simulink model "FinalHTTRModel"  (R2025b)
settings: Solver=ode15s  StartTime=0.0  StopTime=250  MaxStep=0.01  RelTol=1e-3
settings Model: Creator=jf923  LastModifiedBy=dm1124
settings DebuggingCC: AlgebraicLoopMsg=none

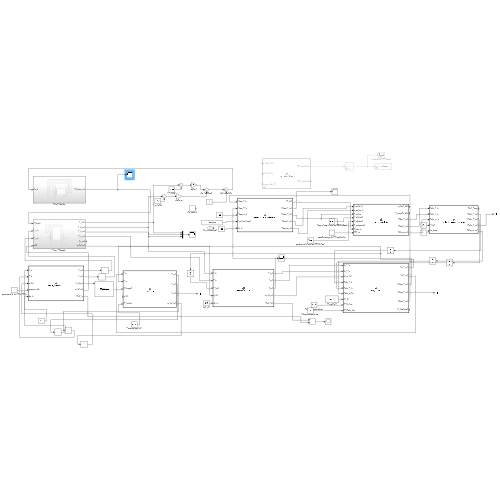
[thumbnail: Simulink's stored preview of the top-level diagram]
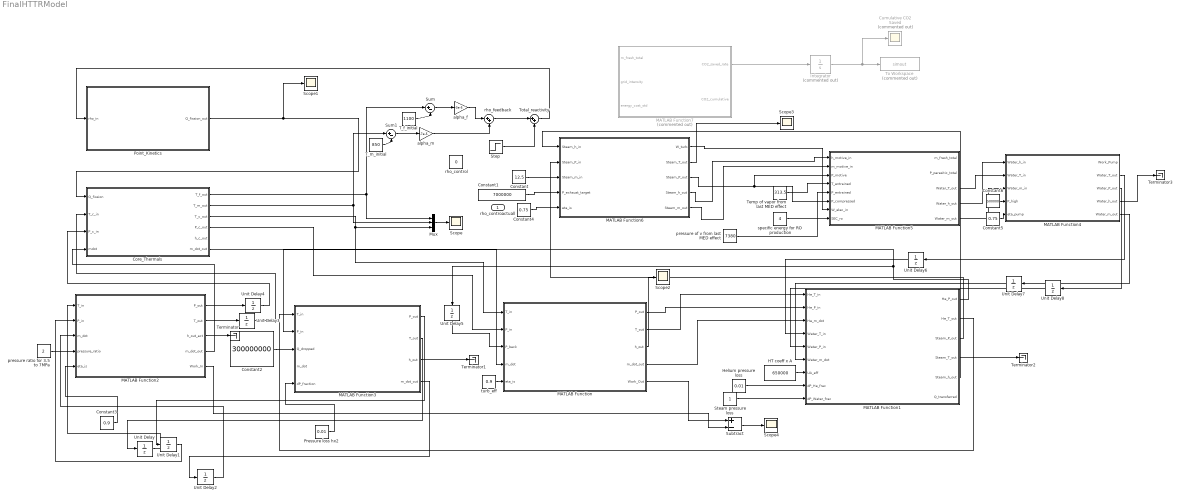
== system FinalHTTRModel ==
  rho_controactuall : Inport
  Constant : Constant  Value=12.5
  Constant1 : Constant  Value=7000000
  Constant2 : Constant  Value=300000000
  Constant3 : Constant  Value=0.9
  Constant4 : Constant  Value=0.75
  Constant5 : Constant  Value=0.75
  Constant6 : Constant  Value=500000
  Core_Thermals : Subsystem
  Cumulative CO2 Saved : Scope  Commented=on
      settings: DataLoggingVariableName=ScopeData3
  HT coeff x A : Constant  Value=650000
  Helium pressure loss : Constant  Value=0.01
  Integrator : Integrator  Commented=on
  MATLAB Function : MATLAB Function  TreatAsAtomicUnit=on  SystemSampleTime=0.1
  MATLAB Function1 : MATLAB Function  TreatAsAtomicUnit=on  SystemSampleTime=0.01
  MATLAB Function2 : MATLAB Function  TreatAsAtomicUnit=on
  MATLAB Function3 : MATLAB Function  TreatAsAtomicUnit=on
  MATLAB Function4 : MATLAB Function  TreatAsAtomicUnit=on
  MATLAB Function5 : MATLAB Function  TreatAsAtomicUnit=on
  MATLAB Function6 : MATLAB Function  TreatAsAtomicUnit=on
  MATLAB Function7 : MATLAB Function  Commented=on  TreatAsAtomicUnit=on
  Mux : Mux  Inputs=3
  Point_Kinetics : Subsystem
  Pressure loss hx2 : Constant  Value=0.01
  Scope{,1..4} (5 alike) : Scope
      Scope settings: ActiveDisplayYMinimum=-2.493928501622884  ActiveDisplayYMaximum=3.810317674067397
      Scope1 settings: ActiveDisplayYMinimum=-6.0368369547673821E+8  ActiveDisplayYMaximum=1.471994974635426E+9
      Scope2 settings: ActiveDisplayYMinimum=2.3690004673826769E+6  ActiveDisplayYMaximum=7.514541427479011E+6  DataLoggingVariableName=ScopeData2
      Scope3 settings: ActiveDisplayYMinimum=344.58792109090257  ActiveDisplayYMaximum=344.7374195032  DataLoggingVariableName=ScopeData5
      Scope4 settings: ActiveDisplayYMinimum=-1.4989347096918812E+9  ActiveDisplayYMaximum=2.98594671527647E+9  DataLoggingVariableName=ScopeData4
  Steam pressure loss : Constant
  Step : Step  Time=100  After=0.001  SampleTime=0
  Subtract : Sum  Inputs=+-
  Sum : Sum  Inputs=|+-
  Sum1 : Sum  Inputs=|+-
  T_f_initial : Constant  Value=1100
  T_m_initial : Constant  Value=850
  Temp of vapor from last MED effect : Constant  Value=313.5
  Terminator{,1..3} (4 alike) : Terminator
  To Workspace : ToWorkspace  Commented=on  VariableName=simout  SaveFormat=Timeseries  SampleTime=-1
  Total_reactivity : Sum  Inputs=|++
  Unit Delay : UnitDelay  InitialCondition=300  SampleTime=-1  HasFrameUpgradeWarning=on
  Unit Delay1 : UnitDelay  InitialCondition=3.5e6  SampleTime=-1  HasFrameUpgradeWarning=on
  Unit Delay2 : UnitDelay  InitialCondition=1000  SampleTime=-1  HasFrameUpgradeWarning=on
  Unit Delay3 : UnitDelay  InitialCondition=500  SampleTime=-1  HasFrameUpgradeWarning=on
  Unit Delay4 : UnitDelay  InitialCondition=7000000  SampleTime=0.01  HasFrameUpgradeWarning=on
  Unit Delay5 : UnitDelay  InitialCondition=7000000  SampleTime=-1  HasFrameUpgradeWarning=on
  Unit Delay6 : UnitDelay  InitialCondition=343  SampleTime=-1  HasFrameUpgradeWarning=on
  Unit Delay7 : UnitDelay  InitialCondition=100  SampleTime=-1  HasFrameUpgradeWarning=on
  Unit Delay8 : UnitDelay  InitialCondition=7000000  SampleTime=-1  HasFrameUpgradeWarning=on
  alpha_f : Gain  Gain=-3e-5
  alpha_m : Gain  Gain=-7e-5
  pressure of v from last MED effect : Constant  Value=7380
  pressure ratio for 3.5 to 7MPa : Constant  Value=2
  rho_control : Constant  Value=0
  rho_feedback : Sum  Inputs=|++
  specific energy for RO production : Constant  Value=4
  turb_eff : Constant  Value=0.9
  wires:
  Point_Kinetics/1(Q_fission_out) -> Core_Thermals/1(Q_fission), Scope1/1
  MATLAB Function/2(T_out) -> MATLAB Function1/1(He_T_in)
  Core_Thermals/1(T_f_out) -> Mux/1, Sum/1
  Core_Thermals/2(T_m_out) -> Mux/2, Sum1/1
  Core_Thermals/3(T_c_out) -> MATLAB Function/1(T_in), Mux/3
  T_f_initial/1 -> Sum/2
  T_m_initial/1 -> Sum1/2
  Sum/1 -> alpha_f/1
  Sum1/1 -> alpha_m/1
  alpha_f/1 -> rho_feedback/1
  alpha_m/1 -> rho_feedback/2
  rho_feedback/1 -> Total_reactivity/1
  Total_reactivity/1 -> Point_Kinetics/1(rho_in)
  Mux/1 -> Scope/1
  Step/1 -> Total_reactivity/2
  turb_eff/1 -> MATLAB Function/5(eta_is)
  MATLAB Function/3(h_out) -> Scope2/1
  MATLAB Function/1(P_out) -> MATLAB Function1/2(He_P_in)
  MATLAB Function/4(m_dot_out) -> MATLAB Function1/3(He_m_dot)
  MATLAB Function2/1(P_out) -> Unit Delay4/1
  Core_Thermals/4(P_c_out) -> MATLAB Function/2(P_in)
  MATLAB Function2/4(m_dot_out) -> Core_Thermals/4(mdot)
  MATLAB Function2/2(T_out) -> Unit Delay3/1
  Core_Thermals/6(m_dot_out) -> MATLAB Function/4(m_dot)
  MATLAB Function1/1(He_P_out) -> MATLAB Function3/2(P_in), Unit Delay5/1
  MATLAB Function1/2(He_T_out) -> MATLAB Function3/1(T_in)
  MATLAB Function1/5(Steam_h_out) -> MATLAB Function6/1(Steam_h_in)
  Constant3/1 -> MATLAB Function2/5(eta_is)
  Helium pressure loss/1 -> MATLAB Function1/8(dP_He_frac)
  MATLAB Function2/5(Work_In) -> Subtract/2
  MATLAB Function/5(Work_Out) -> Subtract/1
  Subtract/1 -> Scope4/1
  MATLAB Function2/3(h_out_act) -> Terminator/1
  MATLAB Function3/3(h_out) -> Terminator1/1
  MATLAB Function1/4(Steam_T_out) -> Terminator2/1
  Constant2/1 -> MATLAB Function3/3(Q_dropped)
  Pressure loss hx2/1 -> MATLAB Function3/5(dP_fraction)
  pressure ratio for 3.5 to 7MPa/1 -> MATLAB Function2/4(pressure_ratio)
  MATLAB Function3/2(T_out) -> Unit Delay/1
  Unit Delay/1 -> MATLAB Function2/1(T_in)
  MATLAB Function3/1(P_out) -> Unit Delay1/1
  MATLAB Function3/4(m_dot_out) -> Unit Delay2/1
  Unit Delay1/1 -> MATLAB Function2/2(P_in)
  Unit Delay2/1 -> MATLAB Function2/3(m_dot)
  Unit Delay3/1 -> Core_Thermals/2(T_c_in)
  Unit Delay4/1 -> Core_Thermals/3(P_c_in)
  Unit Delay5/1 -> MATLAB Function/3(P_back)
  MATLAB Function7/1(CO2_saved_rate) -> Integrator/1
  HT coeff x A/1 -> MATLAB Function1/7(UA_eff)
  Steam pressure loss/1 -> MATLAB Function1/9(dP_Water_frac)
  MATLAB Function5/3(Water_T_out) -> MATLAB Function4/2(Water_T_in)
  MATLAB Function5/5(Water_m_out) -> MATLAB Function4/3(Water_m_in)
  MATLAB Function1/3(Steam_P_out) -> MATLAB Function6/2(Steam_P_in)
  MATLAB Function6/4(Steam_h_out) -> MATLAB Function5/1(h_motive_in)
  MATLAB Function6/5(Steam_m_out) -> MATLAB Function5/2(m_motive_in)
  MATLAB Function6/1(W_turb) -> MATLAB Function5/7(W_elec_in)
  MATLAB Function6/3(Steam_P_out) -> MATLAB Function5/6(P_compressed), MATLAB Function5/3(P_motive)
  Temp of vapor from last MED effect/1 -> MATLAB Function5/4(T_entrained)
  pressure of v from last MED effect/1 -> MATLAB Function5/5(P_entrained)
  specific energy for RO production/1 -> MATLAB Function5/8(SEC_ro)
  MATLAB Function4/3(Water_P_out) -> Unit Delay8/1
  MATLAB Function5/4(Water_h_out) -> MATLAB Function4/1(Water_h_in)
  MATLAB Function4/4(Water_h_out) -> Terminator3/1
  MATLAB Function4/2(Water_T_out) -> Unit Delay6/1
  MATLAB Function4/5(Water_m_out) -> Unit Delay7/1
  Integrator/1 -> Cumulative CO2 Saved/1, To Workspace/1
  Unit Delay6/1 -> MATLAB Function1/4(Water_T_in)
  Unit Delay7/1 -> MATLAB Function1/6(Water_m_dot)
  Unit Delay8/1 -> MATLAB Function1/5(Water_P_in)
  Constant/1 -> MATLAB Function6/3(Steam_m_in)
  Constant1/1 -> MATLAB Function6/4(P_exhaust_target)
  Constant4/1 -> MATLAB Function6/5(eta_is)
  Constant5/1 -> MATLAB Function4/5(eta_pump)
  Constant6/1 -> MATLAB Function4/4(P_high)
  MATLAB Function6/2(Steam_T_out) -> Scope3/1

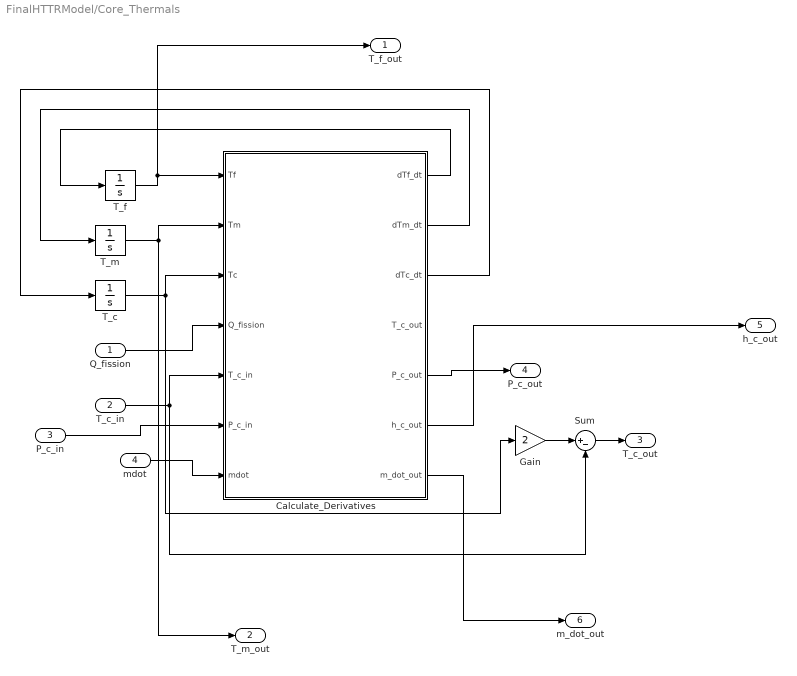
== system FinalHTTRModel/Core_Thermals ==
  Q_fission : Inport
  T_c_in : Inport  Port=2
  P_c_in : Inport  Port=3
  mdot : Inport  Port=4
  Calculate_Derivatives : MATLAB Function  TreatAsAtomicUnit=on
  Gain : Gain  Gain=2
  Sum : Sum  Inputs=|+-
  T_c : Integrator  InitialCondition=550
  T_f : Integrator  InitialCondition=600
  T_m : Integrator  InitialCondition=600
  T_f_out : Outport
  T_m_out : Outport  Port=2
  T_c_out : Outport  Port=3
  P_c_out : Outport  Port=4
  h_c_out : Outport  Port=5
  m_dot_out : Outport  Port=6
  wires:
  T_f/1 -> T_f_out/1, Calculate_Derivatives/1(Tf)
  T_m/1 -> T_m_out/1, Calculate_Derivatives/2(Tm)
  T_c/1 -> Gain/1, Calculate_Derivatives/3(Tc)
  Calculate_Derivatives/1(dTf_dt) -> T_f/1
  Q_fission/1 -> Calculate_Derivatives/4(Q_fission)
  T_c_in/1 -> Sum/2, Calculate_Derivatives/5(T_c_in)
  mdot/1 -> Calculate_Derivatives/7(mdot)
  Gain/1 -> Sum/1
  Sum/1 -> T_c_out/1
  Calculate_Derivatives/2(dTm_dt) -> T_m/1
  Calculate_Derivatives/3(dTc_dt) -> T_c/1
  P_c_in/1 -> Calculate_Derivatives/6(P_c_in)
  Calculate_Derivatives/5(P_c_out) -> P_c_out/1
  Calculate_Derivatives/6(h_c_out) -> h_c_out/1
  Calculate_Derivatives/7(m_dot_out) -> m_dot_out/1

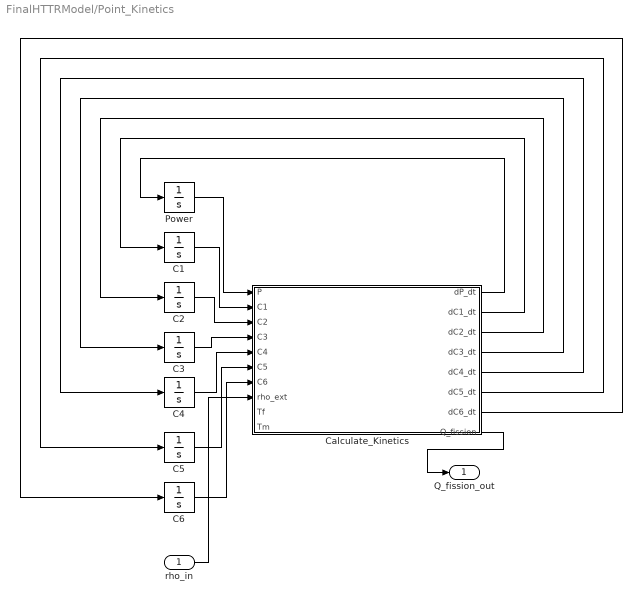
== system FinalHTTRModel/Point_Kinetics ==
  rho_in : Inport
  C1 : Integrator  InitialCondition=32.6371
  C2 : Integrator  InitialCondition=48.8496
  C3 : Integrator  InitialCondition=19.8245
  C4 : Integrator  InitialCondition=16.2791
  C5 : Integrator  InitialCondition=3.1685
  C6 : Integrator  InitialCondition=0.2093
  Calculate_Kinetics : MATLAB Function  TreatAsAtomicUnit=on
  Power : Integrator  InitialCondition=1
  Q_fission_out : Outport
  wires:
  Power/1 -> Calculate_Kinetics/1(P)
  C1/1 -> Calculate_Kinetics/2(C1)
  C2/1 -> Calculate_Kinetics/3(C2)
  C3/1 -> Calculate_Kinetics/4(C3)
  C4/1 -> Calculate_Kinetics/5(C4)
  C5/1 -> Calculate_Kinetics/6(C5)
  C6/1 -> Calculate_Kinetics/7(C6)
  rho_in/1 -> Calculate_Kinetics/8(rho_ext)
  Calculate_Kinetics/1(dP_dt) -> Power/1
  Calculate_Kinetics/2(dC1_dt) -> C1/1
  Calculate_Kinetics/3(dC2_dt) -> C2/1
  Calculate_Kinetics/4(dC3_dt) -> C3/1
  Calculate_Kinetics/5(dC4_dt) -> C4/1
  Calculate_Kinetics/6(dC5_dt) -> C5/1
  Calculate_Kinetics/7(dC6_dt) -> C6/1
  Calculate_Kinetics/8(Q_fission) -> Q_fission_out/1

== matlab function FinalHTTRModel/MATLAB Function2 ==
  data: T_in input; P_out output; T_out output; P_in input; m_dot input; pressure_ratio input; eta_is input; h_out_act output; m_dot_out output; Work_In output
function [P_out, T_out, h_out_act, m_dot_out, Work_In] = helium_compressor(T_in, P_in, m_dot, pressure_ratio, eta_is)
    coder.extrinsic('py.CoolProp.CoolProp.PropsSI');
    P_out = 0.0; T_out = 0.0; h_out_act = 0.0; m_dot_out = 0.0; Work_In = 0.0;
    fluid = 'Helium';
    
    if T_in <= 10 || P_in <= 1000000 || m_dot <= 0
        P_out = double(P_in); T_out = double(T_in); m_dot_out = double(m_dot);
    else
        h_in = 0.0;
        s_in = 0.0;
        h_out_s = 0.0;
        T_out_calc = 0.0;

        h_in_val = py.CoolProp.CoolProp.PropsSI('H', 'T', double(T_in), 'P', double(P_in), fluid);
        h_in = double(h_in_val);
        
        s_in_val = py.CoolProp.CoolProp.PropsSI('S', 'T', double(T_in), 'P', double(P_in), fluid);
        s_in = double(s_in_val);
        
        P_out_target = double(P_in) * double(pressure_ratio);
        
        h_s_val = py.CoolProp.CoolProp.PropsSI('H', 'S', s_in, 'P', P_out_target, fluid);
        h_out_s = double(h_s_val);
        
        h_out_act_val = h_in + (h_out_s - h_in) / double(eta_is);
        h_out_act = double(h_out_act_val);
        
        T_out_val = py.CoolProp.CoolProp.PropsSI('T', 'H', h_out_act, 'P', P_out_target, fluid);
        T_out = double(T_out_val);
        
        P_out = P_out_target;
        m_dot_out = double(m_dot);
        Work_In = double(m_dot) * (h_out_act - h_in);
    end
end

== matlab function FinalHTTRModel/MATLAB Function3 ==
  data: T_in input; P_out output; P_in input; Q_dropped input; m_dot input; dP_fraction input; T_out output; h_out output; m_dot_out output
function [P_out, T_out, h_out, m_dot_out] = helium_hx(T_in, P_in, Q_dropped, m_dot, dP_fraction)
    coder.extrinsic('py.CoolProp.CoolProp.PropsSI');
    P_out = 0.0; T_out = 0.0; h_out = 0.0; m_dot_out = 0.0;
    fluid = 'Helium';
    
    if T_in <= 10 || P_in <= 1000 || m_dot <= 0
        P_out = double(P_in); T_out = double(T_in); m_dot_out = double(m_dot);
    else
        h_in = 0.0;
        T_out_val = 0.0;

        h_in_raw = py.CoolProp.CoolProp.PropsSI('H', 'T', double(T_in), 'P', double(P_in), fluid);
        h_in = double(h_in_raw);
        
        h_out = h_in - (double(Q_dropped) / double(m_dot));
        
        P_out = double(P_in) * (1.0 - double(dP_fraction));
        
        T_out_raw = py.CoolProp.CoolProp.PropsSI('T', 'H', h_out, 'P', P_out, fluid);
        T_out = double(T_out_raw);
        
        m_dot_out = double(m_dot);
    end
end

== matlab function FinalHTTRModel/MATLAB Function4 ==
  data: Work_Pump output; Water_h_in input; Water_T_in input; Water_T_out output; Water_m_in input; P_high input; eta_pump input; Water_P_out output; Water_h_out output; Water_m_out output
function [Work_Pump, Water_T_out, Water_P_out, Water_h_out, Water_m_out] = feedwater_pump_measured(Water_h_in, Water_T_in, Water_m_in, P_high, eta_pump)
    % Declare extrinsic functions for CoolProp
    coder.extrinsic('py.CoolProp.CoolProp.PropsSI');
    fluid = 'Water';
    
    % 1. Pre-initialize variables as doubles to satisfy the Coder
    rho_water = 0.0;
    Work_Pump = 0.0;
    Water_h_out = 0.0;
    Water_T_out = 0.0;
    
    % 2. Calculate Density based on incoming temperature
    % Use an intermediate variable for the mxArray before casting to double
    rho_mx = py.CoolProp.CoolProp.PropsSI('D', 'T', double(Water_T_in), 'P', 31000, fluid);
    rho_water = double(rho_mx);
    
    % 3. Pressurization and Work calculation
    delta_P = double(P_high) - 31000;
    % Ensure all components are treated as numeric doubles
    Work_Pump = (double(Water_m_in) * delta_P) / (rho_water * double(eta_pump));
    
    % 4. Outlet State Assignment
    Water_P_out = double(P_high);
    Water_m_out = double(Water_m_in);
    
    % 5. Calculate Enthalpy increase
    % Work_Pump is now a confirmed double, allowing math operations
    Water_h_out = double(Water_h_in) + (Work_Pump / double(Water_m_in));
    
    % Final CoolProp call for temperature
    T_out_mx = py.CoolProp.CoolProp.PropsSI('T', 'H', Water_h_out, 'P', Water_P_out, fluid);
    Water_T_out = double(T_out_mx);
end

== matlab function FinalHTTRModel/MATLAB Function5 ==
  data: h_motive_in input; m_fresh_total output; m_motive_in input; P_motive input; T_entrained input; P_entrained input; P_compressed input; W_elec_in input; SEC_ro input; P_parasitic_total output; Water_T_out output; Water_h_out output; Water_m_out output
function [m_fresh_total, P_parasitic_total, Water_T_out, Water_h_out, Water_m_out] = hybrid_desal_tvc(h_motive_in, m_motive_in, P_motive, T_entrained, P_entrained, P_compressed, W_elec_in, SEC_ro)
    % h_motive_in: Enthalpy from LP Turbine outlet (Motive Steam)
    % m_motive_in: Steam flow from Turbine (kg/s)
    % T_entrained/P_entrained: Conditions of vapor from last MED effect
    
    coder.extrinsic('py.CoolProp.CoolProp.PropsSI');
    
    Water_h_out = 0;
    % 1. TVC Entrainment Ratio (Ra)
    % Ra = flow rate of motive steam / flow rate of entrained vapor
    % Using the Power (1994) simplified correlation provided in text
    PCF = 3e-7 * P_motive + 0.95; % Pressure Correction Factor
    TCF = 1.0; % Temp Correction Factor (Simplified for Phase 1)
    Cr = P_compressed / P_entrained; % Compression Ratio
    
    % Ra calculation (Semi-empirical model)
    Ra = 0.29 * (Cr^1.19) / (PCF * TCF); 
    m_entrained = m_motive_in / Ra;
    
    % 2. MED Performance (Thermal)
    % Total heating steam = motive + entrained
    m_heating_steam = m_motive_in + m_entrained;
    % GOR is typically higher for TVC (e.g., 10-14)
    GOR_tvc = 12.0; 
    m_fresh_med = m_heating_steam * GOR_tvc; 

    % 3. RO Process (Electrical)
    m_fresh_ro = W_elec_in / (SEC_ro * 3600); % J/kg conversion

    % 4. Output State for Closed-Loop (To Pump/HRSG)
    % The motive steam and entrained vapor condense into liquid water
    Water_m_out = m_motive_in; % Mass balance of the loop fluid
    Water_T_out = 343.15; % 70 C return temp (saturated liquid)
    Water_h_out = double(py.CoolProp.CoolProp.PropsSI('H', 'T', Water_T_out, 'P', P_compressed, 'Water'));
    
    % 5. System Totals
    m_fresh_total = m_fresh_med + m_fresh_ro;
    P_parasitic_total = W_elec_in; % Load for RO Pumps
end

== matlab function FinalHTTRModel/MATLAB Function6 ==
  data: Steam_h_in input; W_turb output; Steam_P_in input; Steam_m_in input; P_exhaust_target input; eta_is input; Steam_T_out output; Steam_P_out output; Steam_h_out output; Steam_m_out output
function [W_turb, Steam_T_out, Steam_P_out, Steam_h_out, Steam_m_out] = steam_turbine_measured(Steam_h_in, Steam_P_in, Steam_m_in, P_exhaust_target, eta_is)
    % Declare extrinsic functions
    coder.extrinsic('py.CoolProp.CoolProp.PropsSI');
    
    % 1. Initialize variables to define them as double scalars for the Coder
    fluid = 'Water';
    s_in = 0; 
    h_out_s = 0;
    T_out_val = 0;
    Steam_T_out = 0;
    
    % 2. Inlet Entropy calculation
    % We call the function and immediately cast the output to double
    s_in_mx = py.CoolProp.CoolProp.PropsSI('S', 'H', double(Steam_h_in), 'P', double(Steam_P_in), fluid);
    s_in = double(s_in_mx); 
    
    % 3. Actual Expansion logic
    % Get isentropic enthalpy
    h_out_s_mx = py.CoolProp.CoolProp.PropsSI('H', 'S', s_in, 'P', double(P_exhaust_target), fluid);
    h_out_s = double(h_out_s_mx);
    
    % Now h_out_s is a native double and can be used in this expression:
    h_out_act = double(Steam_h_in) - (double(eta_is) * (double(Steam_h_in) - h_out_s));
    
    % 4. Outputs
    W_turb = double(Steam_m_in) * (double(Steam_h_in) - h_out_act); % Power in Watts
    Steam_h_out = h_out_act;
    Steam_P_out = double(P_exhaust_target);
    
    % Final temperature calculation
    T_out_mx = py.CoolProp.CoolProp.PropsSI('T', 'H', h_out_act, 'P', double(P_exhaust_target), fluid);
    Steam_T_out = double(T_out_mx);
    
    Steam_m_out = double(Steam_m_in); 
end

== matlab function FinalHTTRModel/MATLAB Function7 ==
  data: m_fresh_total input; CO2_saved_rate output; grid_intensity input; energy_cost_std input; CO2_cumulative output
function [CO2_saved_rate, CO2_cumulative] = co2_offset_logic(m_fresh_total, grid_intensity, energy_cost_std)
    % m_fresh_total: Freshwater produced (kg/s)
    % grid_intensity: kg CO2 emitted per kWh on standard grid (e.g., 0.45)
    % energy_cost_std: kWh required to produce 1 m^3 of water (e.g., 4.0)

    % 1. Convert kg/s of water to m^3/hr
    % (m_fresh_total kg/s) * (3600 s/hr) / (1000 kg/m^3)
    water_m3_hr = (m_fresh_total * 3600) / 1000;

    % 2. Calculate CO2 saved per hour
    % (m^3/hr) * (kWh/m^3) * (kg CO2/kWh) = kg CO2 saved per hour
    CO2_saved_per_hr = water_m3_hr * energy_cost_std * grid_intensity;

    % 3. Output rate in kg/s for the simulation
    CO2_saved_rate = CO2_saved_per_hr / 3600;

    % 4. Cumulative Calculation (Integrated over time)
    % In Simulink, you would typically use an 'Integrator' block 
    % outside of this function to get total kg saved over the run.
    CO2_cumulative = 0; % Placeholder for logic handled by external Integrator
end

== matlab function FinalHTTRModel/Point_Kinetics/Calculate_Kinetics ==
  data: P input; dP_dt output; C1 input; C2 input; C3 input; C4 input; C5 input; C6 input; rho_ext input; dC1_dt output; dC2_dt output; dC3_dt output; dC4_dt output; dC5_dt output; dC6_dt output; Q_fission output; Tf input; Tm input
function [dP_dt, dC1_dt, dC2_dt, dC3_dt, dC4_dt, dC5_dt, dC6_dt, Q_fission] = ...
    Calculate_Kinetics_Final(P, C1, C2, C3, C4, C5, C6, rho_ext, Tf, Tm)
% =========================================================================
% 1. CORE CONSTANTS
% =========================================================================
% 6-Group Delayed Neutron Data for U-235
beta_i = [0.00025, 0.00138, 0.00122, 0.00266, 0.00164, 0.00035];
beta_total = sum(beta_i); 
lambda = [0.0766, 0.2825, 0.6154, 1.634, 5.176, 16.72];
Lambda = 1.0e-3; % Prompt neutron lifetime (s)
Q_nominal = 300e6; % 300 MW thermal nominal power

% --- Feedback Coefficients ---
alpha_f = -3.5e-5; % Fuel temp coefficient
alpha_m = -0.5e-5; % Moderator temp coefficient
Tf_ref = 800;      % Reference Fuel Temp (K)
Tm_ref = 700;      % Reference Moderator Temp (K)

% =========================================================================
% 2. PHYSICAL BOUNDS (PREVENT SINGULARITIES)
% =========================================================================
% Clamp power to reasonable range
P_min = 1e-6;      % Minimum power (prevent zero/negative)
P_max = 10;        % Maximum power (10x nominal = 3000 MW)
P = max(P_min, min(P, P_max));

% Clamp precursor concentrations (must be >= 0)
C1 = max(0, C1); C2 = max(0, C2); C3 = max(0, C3);
C4 = max(0, C4); C5 = max(0, C5); C6 = max(0, C6);

% Clamp temperatures to physical range
Tf = max(300, min(Tf, 2000));  % 300K to 2000K
Tm = max(300, min(Tm, 1500));  % 300K to 1500K

% =========================================================================
% 3. REACTIVITY COUPLING WITH SAFETY LIMITS
% =========================================================================
% Total Reactivity = External (Control Rods) + Internal Feedback
rho_feedback = alpha_f * (Tf - Tf_ref) + alpha_m * (Tm - Tm_ref);
rho_total = rho_ext + rho_feedback;

% **CRITICAL**: Prevent prompt criticality
rho_max = 0.90 * beta_total;  % Never exceed 90% of beta
rho_min = -0.10;              % Maximum shutdown reactivity
rho_total = max(rho_min, min(rho_total, rho_max));

% =========================================================================
% 4. DIFFERENTIAL EQUATIONS (Point Kinetics)
% =========================================================================
% Neutron Population (Power) Derivative
sum_lambda_C = sum(lambda .* [C1, C2, C3, C4, C5, C6]);
dP_dt = ((rho_total - beta_total) / Lambda) * P + sum_lambda_C;

% Precursor Group Derivatives
dC_vec = (beta_i ./ Lambda) .* P - lambda .* [C1, C2, C3, C4, C5, C6];
dC1_dt = dC_vec(1); dC2_dt = dC_vec(2); dC3_dt = dC_vec(3);
dC4_dt = dC_vec(4); dC5_dt = dC_vec(5); dC6_dt = dC_vec(6);

% =========================================================================
% 5. FINAL OUTPUT TO CORE THERMALS
% =========================================================================
Q_fission = P * Q_nominal; % Scaled Power in Watts

end

== matlab function FinalHTTRModel/Core_Thermals/Calculate_Derivatives ==
  data: Tf input; dTf_dt output; dTm_dt output; dTc_dt output; Tm input; Tc input; Q_fission input; T_c_in input; P_c_in input; mdot input; T_c_out output; P_c_out output; h_c_out output; m_dot_out output
function [dTf_dt, dTm_dt, dTc_dt, T_c_out, P_c_out, h_c_out, m_dot_out] = core_thermals(Tf, Tm, Tc, Q_fission, T_c_in, P_c_in, mdot)
    coder.extrinsic('py.CoolProp.CoolProp.PropsSI');
    
    dTf_dt = 0.0; dTm_dt = 0.0; dTc_dt = 0.0; 
    T_c_out = 0.0; P_c_out = 0.0; h_c_out = 0.0; m_dot_out = 0.0;
    fluid = 'Helium';
    
    Cf = 5.0e6; Cm = 1.0e8; Cc = 1.0e6;
    h_fm = 2.0e5; h_fc = 4.0e5; h_mc = 1.5e5;
    
    if T_c_in <= 10 || P_c_in <= 1000 || mdot <= 0
        T_c_out = double(T_c_in);
        P_c_out = double(P_c_in);
        m_dot_out = double(mdot);
    else
        cp_dynamic = 0.0;
        cp_val = py.CoolProp.CoolProp.PropsSI('C', 'T', double(Tc), 'P', double(P_c_in), fluid);
        cp_dynamic = double(cp_val);
        
        dTf_dt = (double(Q_fission) - h_fm*(Tf - Tm) - h_fc*(Tf - Tc)) / Cf;
        dTm_dt = (h_fm*(Tf - Tm) - h_mc*(Tm - Tc)) / Cm;
        
        dTc_dt = (h_fc*(Tf - Tc) + h_mc*(Tm - Tc) - 2.0*double(mdot)*cp_dynamic*(Tc - double(T_c_in))) / Cc;
        
        T_c_out = 2.0*Tc - double(T_c_in);      
        P_c_out = double(P_c_in) * 0.98;     
        
        h_c_out = 0.0;
        h_val = py.CoolProp.CoolProp.PropsSI('H', 'T', T_c_out, 'P', P_c_out, fluid);
        h_c_out = double(h_val);
        m_dot_out = double(mdot);
    end
end

== matlab function FinalHTTRModel/MATLAB Function ==
  data: P_out output; T_in input; T_out output; P_in input; P_back input; m_dot input; h_out output; eta_is input; m_dot_out output; Work_Out output
function [P_out, T_out, h_out, m_dot_out, Work_Out] = helium_turbine(T_in, P_in, P_back, m_dot, eta_is)
    coder.extrinsic('py.CoolProp.CoolProp.PropsSI');
    P_out = 0.0; T_out = 0.0; h_out = 0.0; m_dot_out = 0.0; Work_Out = 0.0;
    fluid = 'Helium';
    if T_in <= 10 || P_in <= 1000 || m_dot <= 0
        P_out = double(P_in); T_out = double(T_in); m_dot_out = double(m_dot);
    else
        % Initialize variables as doubles before extrinsic calls
        h_in = 0.0;
        s_in = 0.0;
        h_out_s = 0.0;
        T_out_val = 0.0;

        h_in = double(py.CoolProp.CoolProp.PropsSI('H', 'T', double(T_in), 'P', double(P_in), fluid));
        s_in = double(py.CoolProp.CoolProp.PropsSI('S', 'T', double(T_in), 'P', double(P_in), fluid));
        
        h_s_val = py.CoolProp.CoolProp.PropsSI('H', 'S', s_in, 'P', double(P_back), fluid);
        h_out_s = double(h_s_val);
        
        h_out_actual = h_in - (double(eta_is) * (h_in - h_out_s));
        h_out = double(h_out_actual);
        
        temp_T = py.CoolProp.CoolProp.PropsSI('T', 'H', h_out, 'P', double(P_back), fluid);
        T_out = double(temp_T);
        
        P_out = double(P_back);
        m_dot_out = double(m_dot);
        Work_Out = double(m_dot) * (h_in - h_out);
    end
end

== matlab function FinalHTTRModel/MATLAB Function1 ==
  data: He_T_in input; He_P_out output; He_P_in input; He_m_dot input; Water_T_in input; Water_P_in input; He_T_out output; Steam_P_out output; Steam_T_out output; Steam_h_out output; Q_transferred output; Water_m_dot input; UA_eff input; dP_He_frac input; dP_Water_frac input
function [He_P_out, He_T_out, Steam_P_out, Steam_T_out, Steam_h_out, Q_transferred] = ...
    hrsg_boiler(He_T_in, He_P_in, He_m_dot, Water_T_in, Water_P_in, Water_m_dot, UA_eff, dP_He_frac, dP_Water_frac)

    % Declare extrinsic for Coder compatibility
    coder.extrinsic('py.CoolProp.CoolProp.PropsSI');
    
    % Strings for CoolProp
    fluid_he = 'Helium';
    fluid_water = 'Water';
    h_he_in = 0;
    h_he_target = 0;
    h_water_in = 0;
    He_T_out =0;
    Steam_T_out=0;

    

    % Fluids
    fluid_he    = 'Helium';
    fluid_water = 'Water';

    %% ---------------- 1. INPUT SAFETY ----------------

    % Helium
    T_he_safe = double(He_T_in);
    if T_he_safe < 100
        T_he_safe = 1000;
    end

    P_he_safe = double(He_P_in);
    if P_he_safe < 1e3
        P_he_safe = 7e6;
    end

    m_dot_he_safe = double(He_m_dot);
    if m_dot_he_safe < 1e-3
        m_dot_he_safe = 85.0;
    end

    % Water
    T_water_safe = double(Water_T_in);
    if T_water_safe < 200
        T_water_safe = 343.15;
    end

    P_water_safe = double(Water_P_in);
    if P_water_safe < 1e3
        P_water_safe = 7e6;
    end

    m_dot_water_safe = double(Water_m_dot);
    if m_dot_water_safe < 1e-3
        m_dot_water_safe = 100.0;
    end

    %% ---------------- 2. CLAMP PRESSURE DROPS ----------------

    dP_He = min(max(double(dP_He_frac),    0.0), 0.9);
    dP_W  = min(max(double(dP_Water_frac), 0.0), 0.9);

    %% ---------------- 3. THERMODYNAMICS ----------------

    % Helium inlet enthalpy
    h_he_in = double(py.CoolProp.CoolProp.PropsSI( ...
        'H','T',T_he_safe,'P',P_he_safe,fluid_he));

    % Helium target enthalpy (672 K)
    h_he_target = double(py.CoolProp.CoolProp.PropsSI( ...
        'H','T',672.0,'P',P_he_safe,fluid_he));

    % Heat transfer
    Q_transferred = m_dot_he_safe * (h_he_in - h_he_target);

    % Water inlet enthalpy
    h_water_in = double(py.CoolProp.CoolProp.PropsSI( ...
        'H','T',T_water_safe,'P',P_water_safe,fluid_water));

    %% ---------------- 4. OUTLET STATES ----------------

    % Helium outlet
    He_P_out = P_he_safe * (1.0 - dP_He);
    if He_P_out < 1e3
        He_P_out = 1e5;
    end

    h_he_out = h_he_in - Q_transferred / m_dot_he_safe;

    % Steam outlet
    Steam_P_out = P_water_safe * (1.0 - dP_W);
    if Steam_P_out < 1e3
        Steam_P_out = 1e5;
    end

    h_steam_out = h_water_in + Q_transferred / m_dot_water_safe;

    % Enthalpy sanity
    if h_steam_out < 1e5
        h_steam_out = 3e5;
    end

    Steam_h_out = h_steam_out;

    %% ---------------- 5. FINAL TEMPERATURE LOOKUPS ----------------

    He_T_out = double(py.CoolProp.CoolProp.PropsSI( ...
        'T','H',h_he_out,'P',He_P_out,fluid_he));

    Steam_T_out = double(py.CoolProp.CoolProp.PropsSI( ...
        'T','H',h_steam_out,'P',Steam_P_out,fluid_water));

end
